simulink library "lib_Convection_FCTiltedRectCavity"  (R2015a)
settings: Solver=ode45  StartTime=0.0  StopTime=10.0  RelTol=1e-3
libraries: simulink x1
settings Model: Creator=jlkratz  LastModifiedBy=jlkratz

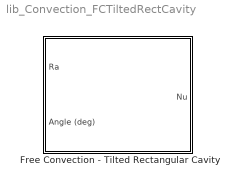
== system lib_Convection_FCTiltedRectCavity ==
  Free Convection - Tilted Rectangular Cavity : Subsystem  mask(TSAT: Tilted Rectangular Cavity){AR_M=[1 12]}
      mask prompts: AR_M "AR_M - Aspect ratio of the rectangular cavity (H/L) where H is the height and L is the distance between the hot and cold walls"
      mask help:
      | This block estimates the average Nusselt number of free convection within a tilted rectangular cavity.  Two opposite surfaces are heated and cooled while the horizontal surfaces are adiabatic. The flow motion is characterized by a combination of recirculating or cellular flow and roll structures. The transitions between these two types of fluid motion typically occurs at a critical tilt angle. Depending on the tilt angle and aspect ratio (H/L), one of variety of correlation is used in the block to approximate the average Nusselt number. Note that all fluid properrties should be evaluated at average of the hot and cold surface. Also note that the charateristic length used to calculate the Rayleigh number should be the distance between the hot and cold surfaces (L).
      |
      | See the help menu for more information.
      mask Help: web(which('Convection_TSAT_FCTiltedRectCavity.html'),'-helpbrowser')

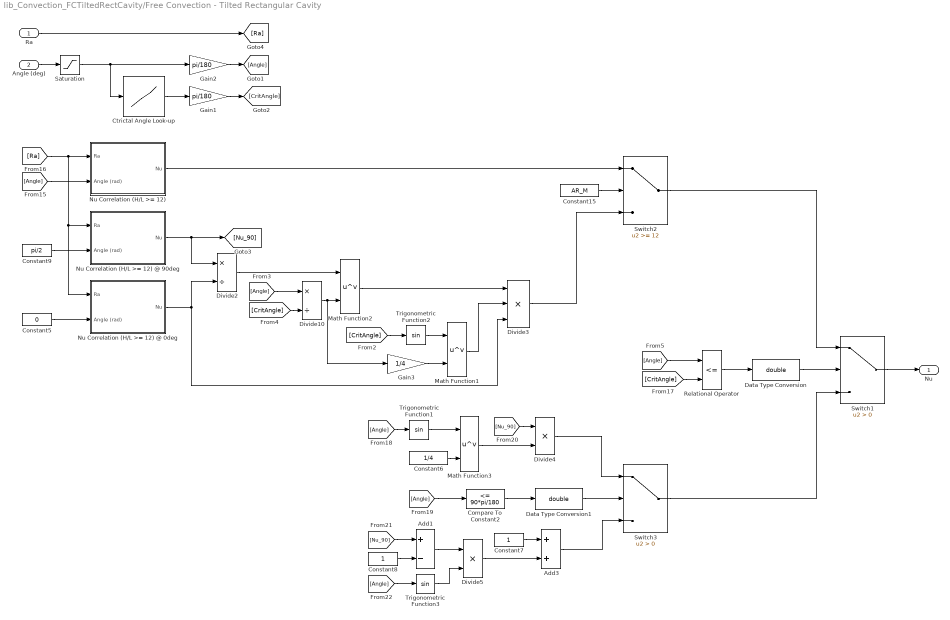
== system lib_Convection_FCTiltedRectCavity/Free Convection - Tilted Rectangular Cavity ==
  Ra : Inport
  Angle (deg) : Inport  Port=2
  Add1 : Sum  Inputs=+-
  Add3 : Sum
  Compare To Constant2 : simulink/Logic and Bit Operations/Compare To Constant  relop=<=  const=90*pi/180  OutDataTypeStr=boolean
  Constant15 : Constant  Value=AR_M
  Constant5 : Constant  Value=0
  Constant6 : Constant  Value=1/4
  Constant7 : Constant
  Constant8 : Constant
  Constant9 : Constant  Value=pi/2
  Ctrictal Angle Look-up : Lookup_n-D  NumberOfTableDimensions=1  BreakpointsForDimension1=[1 3 6 12 15 20]  Table=[25 53 60 67 70 70]  InternalRulePriority=Speed  RndMeth=Simplest  InputSameDT=on
  Data Type Conversion : DataTypeConversion  OutDataTypeStr=double
  Data Type Conversion1 : DataTypeConversion  OutDataTypeStr=double
  Divide10 : Product  Inputs=*/
  Divide2 : Product  Inputs=*/
  Divide3 : Product  Inputs=***
  Divide4 : Product  Inputs=**
  Divide5 : Product  Inputs=**
  Gain1 : Gain  Gain=pi/180
  Gain2 : Gain  Gain=pi/180
  Gain3 : Gain  Gain=1/4
  Math Function1 : Math  Operator=pow  SaturateOnIntegerOverflow=on
  Math Function2 : Math  Operator=pow  SaturateOnIntegerOverflow=on
  Math Function3 : Math  Operator=pow  SaturateOnIntegerOverflow=on
  Nu Correlation (H/L >= 12) : Subsystem
  Nu Correlation (H/L >= 12) @ 0deg : Subsystem
  Nu Correlation (H/L >= 12) @ 90deg : Subsystem
  Relational Operator : RelationalOperator  Operator=<=  OutDataTypeStr=boolean
  Saturation : Saturate  UpperLimit=180  LowerLimit=0
  Switch1 : Switch  Criteria=u2 > Threshold
  Switch2 : Switch  Threshold=12
  Switch3 : Switch  Criteria=u2 > Threshold
  Trigonometric Function1 : Trigonometry
  Trigonometric Function2 : Trigonometry
  Trigonometric Function3 : Trigonometry
  Nu : Outport
  wires:
  Switch2/1 -> Switch1/1
  Switch3/1 -> Switch1/3
  Saturation/1 -> Gain2/1, Ctrictal Angle Look-up/1
  Add3/1 -> Switch3/3
  Divide5/1 -> Add3/2
  Add1/1 -> Divide5/1
  Trigonometric Function3/1 -> Divide5/2
  [Angle] -> Trigonometric Function3/1
  Constant8/1 -> Add1/2
  [Nu_90] -> Add1/1
  Constant7/1 -> Add3/1
  Divide4/1 -> Switch3/1
  Math Function3/1 -> Divide4/2
  [Nu_90] -> Divide4/1
  Constant6/1 -> Math Function3/2
  Trigonometric Function1/1 -> Math Function3/1
  [Angle] -> Trigonometric Function1/1
  Compare To Constant2/1 -> Data Type Conversion1/1
  Data Type Conversion1/1 -> Switch3/2
  [Angle] -> Compare To Constant2/1
  Switch1/1 -> Nu/1
  Data Type Conversion/1 -> Switch1/2
  Relational Operator/1 -> Data Type Conversion/1
  [Angle] -> Relational Operator/1
  [CritAngle] -> Relational Operator/2
  Divide3/1 -> Switch2/3
  Math Function1/1 -> Divide3/2
  Math Function2/1 -> Divide3/1
  Divide10/1 -> Math Function2/2, Gain3/1
  Gain3/1 -> Math Function1/2
  [CritAngle] -> Trigonometric Function2/1
  Divide2/1 -> Math Function2/1
  Nu Correlation (H/L >= 12) @ 0deg/1(Nu) -> Divide2/2, Divide3/3
  Nu Correlation (H/L >= 12) @ 90deg/1(Nu) -> Divide2/1, [Nu_90]
  [Angle] -> Divide10/1
  [CritAngle] -> Divide10/2
  Gain1/1 -> [CritAngle]
  Ctrictal Angle Look-up/1 -> Gain1/1
  Constant5/1 -> Nu Correlation (H/L >= 12) @ 0deg/2(Angle (rad))
  Trigonometric Function2/1 -> Math Function1/1
  Constant9/1 -> Nu Correlation (H/L >= 12) @ 90deg/2(Angle (rad))
  Nu Correlation (H/L >= 12)/1(Nu) -> Switch2/1
  [Angle] -> Nu Correlation (H/L >= 12)/2(Angle (rad))
  [Ra] -> Nu Correlation (H/L >= 12) @ 90deg/1(Ra), Nu Correlation (H/L >= 12) @ 0deg/1(Ra), Nu Correlation (H/L >= 12)/1(Ra)
  Constant15/1 -> Switch2/2
  Gain2/1 -> [Angle]
  Angle (deg)/1 -> Saturation/1
  Ra/1 -> [Ra]

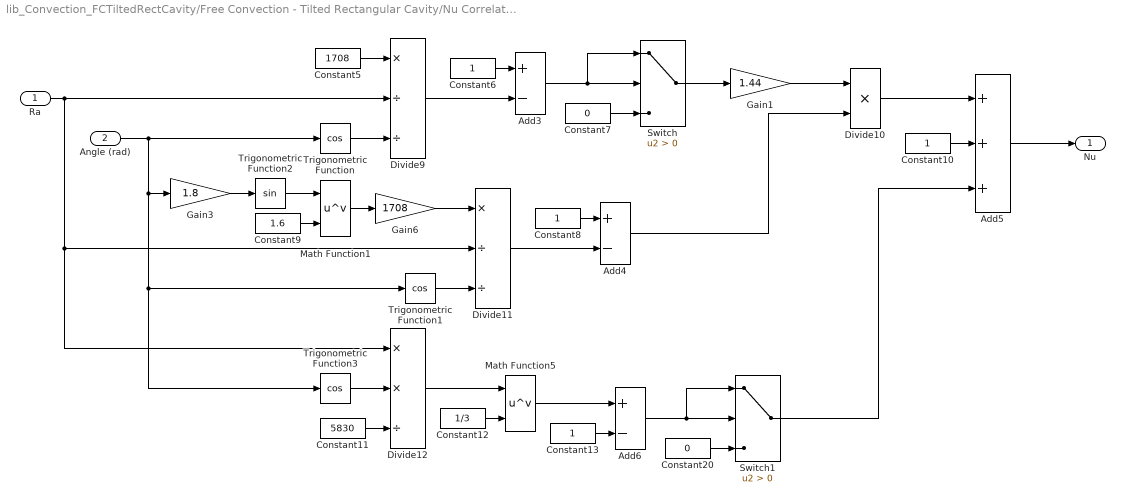
== system lib_Convection_FCTiltedRectCavity/Free Convection - Tilted Rectangular Cavity/Nu Correlation (H//L >= 12) ==
  Ra : Inport
  Angle (rad) : Inport  Port=2
  Add3 : Sum  Inputs=+-
  Add4 : Sum  Inputs=+-
  Add5 : Sum  Inputs=+++
  Add6 : Sum  Inputs=+-
  Constant{6,8,10,13} (4 alike) : Constant
  Constant11 : Constant  Value=5830
  Constant12 : Constant  Value=1/3
  Constant20 : Constant  Value=0
  Constant5 : Constant  Value=1708
  Constant7 : Constant  Value=0
  Constant9 : Constant  Value=1.6
  Divide10 : Product  Inputs=**
  Divide11 : Product  Inputs=*//
  Divide12 : Product  Inputs=**/
  Divide9 : Product  Inputs=*//
  Gain1 : Gain  Gain=1.44
  Gain3 : Gain  Gain=1.8
  Gain6 : Gain  Gain=1708
  Math Function1 : Math  Operator=pow  SaturateOnIntegerOverflow=on
  Math Function5 : Math  Operator=pow  SaturateOnIntegerOverflow=on
  Switch : Switch  Criteria=u2 > Threshold
  Switch1 : Switch  Criteria=u2 > Threshold
  Trigonometric Function : Trigonometry  Operator=cos
  Trigonometric Function1 : Trigonometry  Operator=cos
  Trigonometric Function2 : Trigonometry
  Trigonometric Function3 : Trigonometry  Operator=cos
  Nu : Outport
  wires:
  Constant8/1 -> Add4/1
  Trigonometric Function1/1 -> Divide11/3
  Angle (rad)/1 -> Gain3/1, Trigonometric Function1/1, Trigonometric Function3/1, Trigonometric Function/1
  Divide11/1 -> Add4/2
  Switch/1 -> Gain1/1
  Constant5/1 -> Divide9/1
  Constant10/1 -> Add5/2
  Constant6/1 -> Add3/1
  Ra/1 -> Divide9/2, Divide11/2, Divide12/1
  Constant7/1 -> Switch/3
  Add3/1 -> Switch/2, Switch/1
  Gain3/1 -> Trigonometric Function2/1
  Trigonometric Function2/1 -> Math Function1/1
  Constant9/1 -> Math Function1/2
  Add4/1 -> Divide10/2
  Math Function1/1 -> Gain6/1
  Constant12/1 -> Math Function5/2
  Divide12/1 -> Math Function5/1
  Gain1/1 -> Divide10/1
  Gain6/1 -> Divide11/1
  Trigonometric Function/1 -> Divide9/3
  Divide9/1 -> Add3/2
  Constant13/1 -> Add6/2
  Math Function5/1 -> Add6/1
  Constant11/1 -> Divide12/3
  Add5/1 -> Nu/1
  Switch1/1 -> Add5/3
  Constant20/1 -> Switch1/3
  Add6/1 -> Switch1/2, Switch1/1
  Divide10/1 -> Add5/1
  Trigonometric Function3/1 -> Divide12/2

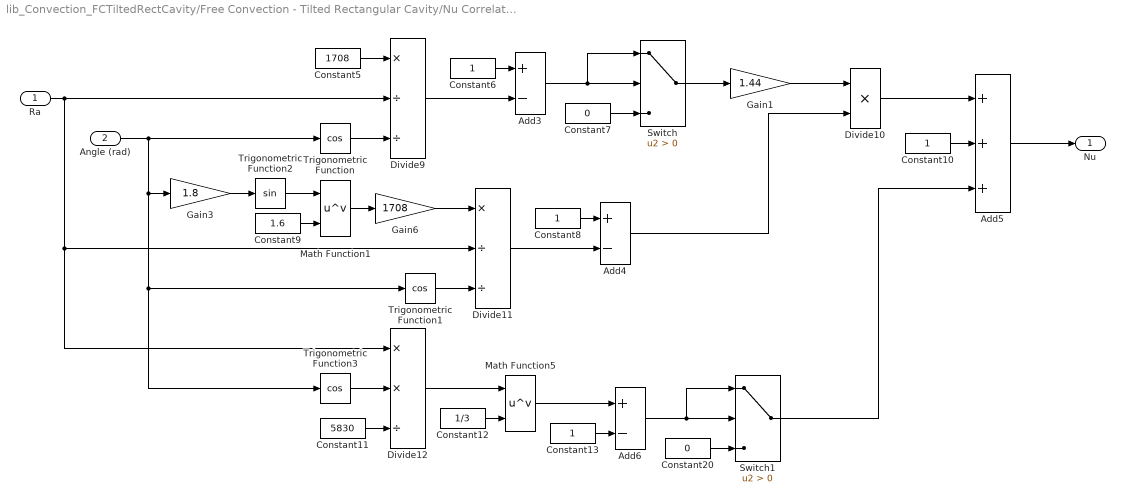
== system lib_Convection_FCTiltedRectCavity/Free Convection - Tilted Rectangular Cavity/Nu Correlation (H//L >= 12) @ 0deg ==
  Ra : Inport
  Angle (rad) : Inport  Port=2
  Add3 : Sum  Inputs=+-
  Add4 : Sum  Inputs=+-
  Add5 : Sum  Inputs=+++
  Add6 : Sum  Inputs=+-
  Constant{6,8,10,13} (4 alike) : Constant
  Constant11 : Constant  Value=5830
  Constant12 : Constant  Value=1/3
  Constant20 : Constant  Value=0
  Constant5 : Constant  Value=1708
  Constant7 : Constant  Value=0
  Constant9 : Constant  Value=1.6
  Divide10 : Product  Inputs=**
  Divide11 : Product  Inputs=*//
  Divide12 : Product  Inputs=**/
  Divide9 : Product  Inputs=*//
  Gain1 : Gain  Gain=1.44
  Gain3 : Gain  Gain=1.8
  Gain6 : Gain  Gain=1708
  Math Function1 : Math  Operator=pow  SaturateOnIntegerOverflow=on
  Math Function5 : Math  Operator=pow  SaturateOnIntegerOverflow=on
  Switch : Switch  Criteria=u2 > Threshold
  Switch1 : Switch  Criteria=u2 > Threshold
  Trigonometric Function : Trigonometry  Operator=cos
  Trigonometric Function1 : Trigonometry  Operator=cos
  Trigonometric Function2 : Trigonometry
  Trigonometric Function3 : Trigonometry  Operator=cos
  Nu : Outport
  wires:
  Constant8/1 -> Add4/1
  Trigonometric Function1/1 -> Divide11/3
  Angle (rad)/1 -> Gain3/1, Trigonometric Function1/1, Trigonometric Function3/1, Trigonometric Function/1
  Divide11/1 -> Add4/2
  Switch/1 -> Gain1/1
  Constant5/1 -> Divide9/1
  Constant10/1 -> Add5/2
  Constant6/1 -> Add3/1
  Ra/1 -> Divide9/2, Divide11/2, Divide12/1
  Constant7/1 -> Switch/3
  Add3/1 -> Switch/2, Switch/1
  Gain3/1 -> Trigonometric Function2/1
  Trigonometric Function2/1 -> Math Function1/1
  Constant9/1 -> Math Function1/2
  Add4/1 -> Divide10/2
  Math Function1/1 -> Gain6/1
  Constant12/1 -> Math Function5/2
  Divide12/1 -> Math Function5/1
  Gain1/1 -> Divide10/1
  Gain6/1 -> Divide11/1
  Trigonometric Function/1 -> Divide9/3
  Divide9/1 -> Add3/2
  Constant13/1 -> Add6/2
  Math Function5/1 -> Add6/1
  Constant11/1 -> Divide12/3
  Add5/1 -> Nu/1
  Switch1/1 -> Add5/3
  Constant20/1 -> Switch1/3
  Add6/1 -> Switch1/2, Switch1/1
  Divide10/1 -> Add5/1
  Trigonometric Function3/1 -> Divide12/2

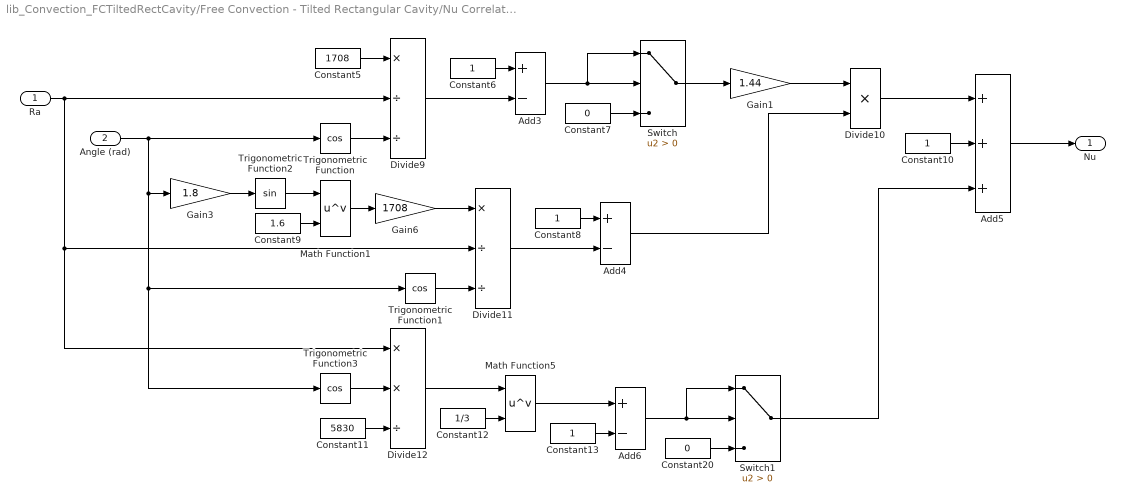
== system lib_Convection_FCTiltedRectCavity/Free Convection - Tilted Rectangular Cavity/Nu Correlation (H//L >= 12) @ 90deg ==
  Ra : Inport
  Angle (rad) : Inport  Port=2
  Add3 : Sum  Inputs=+-
  Add4 : Sum  Inputs=+-
  Add5 : Sum  Inputs=+++
  Add6 : Sum  Inputs=+-
  Constant{6,8,10,13} (4 alike) : Constant
  Constant11 : Constant  Value=5830
  Constant12 : Constant  Value=1/3
  Constant20 : Constant  Value=0
  Constant5 : Constant  Value=1708
  Constant7 : Constant  Value=0
  Constant9 : Constant  Value=1.6
  Divide10 : Product  Inputs=**
  Divide11 : Product  Inputs=*//
  Divide12 : Product  Inputs=**/
  Divide9 : Product  Inputs=*//
  Gain1 : Gain  Gain=1.44
  Gain3 : Gain  Gain=1.8
  Gain6 : Gain  Gain=1708
  Math Function1 : Math  Operator=pow  SaturateOnIntegerOverflow=on
  Math Function5 : Math  Operator=pow  SaturateOnIntegerOverflow=on
  Switch : Switch  Criteria=u2 > Threshold
  Switch1 : Switch  Criteria=u2 > Threshold
  Trigonometric Function : Trigonometry  Operator=cos
  Trigonometric Function1 : Trigonometry  Operator=cos
  Trigonometric Function2 : Trigonometry
  Trigonometric Function3 : Trigonometry  Operator=cos
  Nu : Outport
  wires:
  Trigonometric Function3/1 -> Divide12/2
  Divide10/1 -> Add5/1
  Add6/1 -> Switch1/1, Switch1/2
  Constant20/1 -> Switch1/3
  Switch1/1 -> Add5/3
  Add5/1 -> Nu/1
  Constant11/1 -> Divide12/3
  Math Function5/1 -> Add6/1
  Constant13/1 -> Add6/2
  Divide9/1 -> Add3/2
  Trigonometric Function/1 -> Divide9/3
  Gain6/1 -> Divide11/1
  Gain1/1 -> Divide10/1
  Divide12/1 -> Math Function5/1
  Constant12/1 -> Math Function5/2
  Math Function1/1 -> Gain6/1
  Add4/1 -> Divide10/2
  Constant9/1 -> Math Function1/2
  Trigonometric Function2/1 -> Math Function1/1
  Gain3/1 -> Trigonometric Function2/1
  Add3/1 -> Switch/1, Switch/2
  Constant7/1 -> Switch/3
  Ra/1 -> Divide12/1, Divide11/2, Divide9/2
  Constant6/1 -> Add3/1
  Constant10/1 -> Add5/2
  Constant5/1 -> Divide9/1
  Switch/1 -> Gain1/1
  Divide11/1 -> Add4/2
  Angle (rad)/1 -> Trigonometric Function/1, Trigonometric Function3/1, Trigonometric Function1/1, Gain3/1
  Trigonometric Function1/1 -> Divide11/3
  Constant8/1 -> Add4/1
